simulink model "MdSWReqChk"  (R2024b)
settings: Solver=FixedStepDiscrete  StartTime=0.0  StopTime=10.0  FixedStep=0.01  RelTol=1e-3
undefined symbols (not defined in the file or in its folder): ChkBsyBitArray4s, ChkBsyBitArray6s7s, KeSMSAutoEZEFwdBkwdPosEna_Val, KeSMSuButtonLongPressedThrshldTm_Val, KeSMSuMdNum4s_Val, KeSMSuMdNum6s7s_Val, SetBsyBitArray4s, SetEnBitArray4s
libraries: simulink x16, RspLib x14
(part 3 of 3)

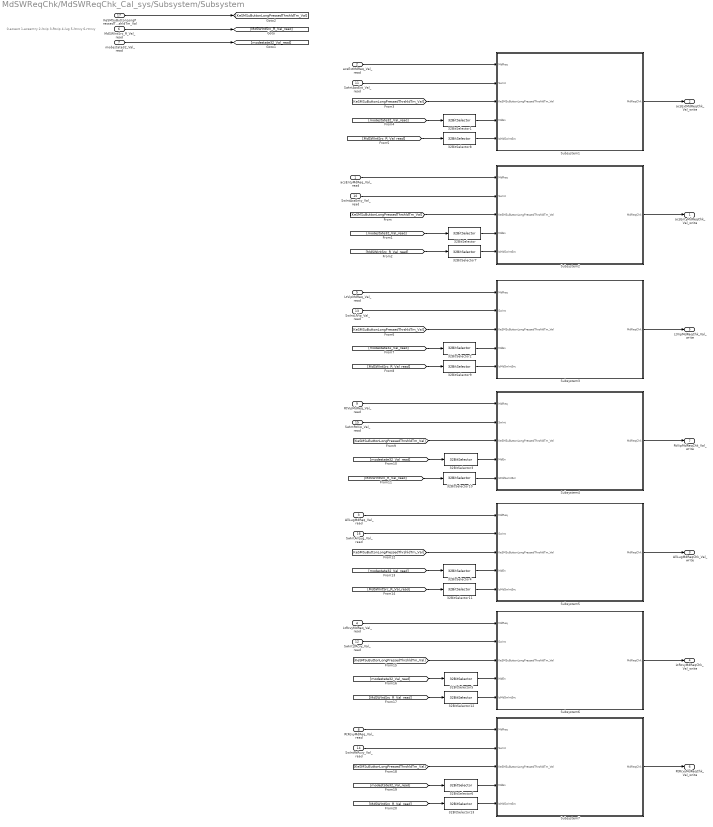
== system MdSWReqChk/MdSWReqChk_Cal_sys/Subsystem/Subsystem ==
  note: 0-acsext 1-acsentry 2-ltvip 3-Rtvip 4-lug 5-ltrcvy 6-rtrcvy
  acsEntyMdReq_Val_read : Inport
  acsExtMdReq_Val_read : Inport  Port=2
  AllLugMdReq_Val_read : Inport  Port=3
  LtRcvyMdReq_Val_read : Inport  Port=4
  LtVipMdReq_Val_read : Inport  Port=5
  MdSWIntSrc_R_Val_read : Inport  Port=6
  modestate32_Val_read : Inport  Port=7
  RtRcvyMdReq_Val_read : Inport  Port=8
  RtVipMdReq_Val_read : Inport  Port=9
  SwIntAcsEnty_Val_read : Inport  Port=10
  SwIntAcsExt_Val_read : Inport  Port=11
  SwIntLfRcvy_Val_read : Inport  Port=12
  SwIntLfVip_Val_read : Inport  Port=13
  SwIntRtRcvy_Val_read : Inport  Port=14
  SwIntRtVip_Val_read : Inport  Port=15
  SwIntAllLug_Val_read : Inport  Port=16
  KeSMSuButtonLongPressedThrshldTm_Val : Inport  Port=17
  32BitSelector : RspLib/32BitSelector  BitNum=0
  32BitSelector1 : RspLib/32BitSelector  BitNum=3
  32BitSelector10 : RspLib/32BitSelector  BitNum=3
  32BitSelector11 : RspLib/32BitSelector  BitNum=4
  32BitSelector12 : RspLib/32BitSelector  BitNum=5
  32BitSelector13 : RspLib/32BitSelector  BitNum=6
  32BitSelector2 : RspLib/32BitSelector  BitNum=9
  32BitSelector3 : RspLib/32BitSelector  BitNum=11
  32BitSelector4 : RspLib/32BitSelector  BitNum=2
  32BitSelector5 : RspLib/32BitSelector  BitNum=10
  32BitSelector6 : RspLib/32BitSelector  BitNum=12
  32BitSelector7 : RspLib/32BitSelector  BitNum=1
  32BitSelector8 : RspLib/32BitSelector  BitNum=0
  32BitSelector9 : RspLib/32BitSelector  BitNum=2
  Subsystem1 : Subsystem
  Subsystem2 : Subsystem
  Subsystem3 : Subsystem
  Subsystem4 : Subsystem
  Subsystem5 : Subsystem
  Subsystem6 : Subsystem
  Subsystem7 : Subsystem
  acsEntyMdReqChk_Val_write : Outport  VectorParamsAs1DForOutWhenUnconnected=off
      settings: EnsureOutportIsVirtual=on
  acsExtMdReqChk_Val_write : Outport  Port=2  VectorParamsAs1DForOutWhenUnconnected=off
      settings: EnsureOutportIsVirtual=on
  AllLugMdReqChk_Val_write : Outport  Port=3  VectorParamsAs1DForOutWhenUnconnected=off
      settings: EnsureOutportIsVirtual=on
  LtRcvyMdReqChk_Val_write : Outport  Port=4  VectorParamsAs1DForOutWhenUnconnected=off
      settings: EnsureOutportIsVirtual=on
  LtVipMdReqChk_Val_write : Outport  Port=5  VectorParamsAs1DForOutWhenUnconnected=off
      settings: EnsureOutportIsVirtual=on
  RtRcvyMdReqChk_Val_write : Outport  Port=6  VectorParamsAs1DForOutWhenUnconnected=off
      settings: EnsureOutportIsVirtual=on
  RtVipMdReqChk_Val_write : Outport  Port=7  VectorParamsAs1DForOutWhenUnconnected=off
      settings: EnsureOutportIsVirtual=on
  wires:
  modestate32_Val_read/1 -> [modestate32_Val_read]
  SwIntAcsExt_Val_read/1 -> Subsystem1/2(SwInt)
  MdSWIntSrc_R_Val_read/1 -> [MdSWIntSrc_R_Val_read]
  SwIntAcsEnty_Val_read/1 -> Subsystem2/2(SwInt)
  KeSMSuButtonLongPressedThrshldTm_Val/1 -> [KeSMSuButtonLongPressedThrshldTm_Val]
  [KeSMSuButtonLongPressedThrshldTm_Val] -> Subsystem2/3(KeSMSuButtonLongPressedThrshldTm_Val)
  [modestate32_Val_read] -> 32BitSelector/1
  32BitSelector/1 -> Subsystem2/4(MdEn)
  [MdSWIntSrc_R_Val_read] -> 32BitSelector7/1
  32BitSelector7/1 -> Subsystem2/5(IsMdSwIntSrc)
  Subsystem2/1(MdReqChk) -> acsEntyMdReqChk_Val_write/1
  [KeSMSuButtonLongPressedThrshldTm_Val] -> Subsystem1/3(KeSMSuButtonLongPressedThrshldTm_Val)
  32BitSelector1/1 -> Subsystem1/4(MdEn)
  [modestate32_Val_read] -> 32BitSelector1/1
  32BitSelector8/1 -> Subsystem1/5(IsMdSwIntSrc)
  [MdSWIntSrc_R_Val_read] -> 32BitSelector8/1
  Subsystem1/1(MdReqChk) -> acsExtMdReqChk_Val_write/1
  acsExtMdReq_Val_read/1 -> Subsystem1/1(MdReq)
  acsEntyMdReq_Val_read/1 -> Subsystem2/1(MdReq)
  32BitSelector2/1 -> Subsystem3/4(MdEn)
  32BitSelector9/1 -> Subsystem3/5(IsMdSwIntSrc)
  [KeSMSuButtonLongPressedThrshldTm_Val] -> Subsystem3/3(KeSMSuButtonLongPressedThrshldTm_Val)
  [modestate32_Val_read] -> 32BitSelector2/1
  32BitSelector3/1 -> Subsystem4/4(MdEn)
  32BitSelector10/1 -> Subsystem4/5(IsMdSwIntSrc)
  [KeSMSuButtonLongPressedThrshldTm_Val] -> Subsystem4/3(KeSMSuButtonLongPressedThrshldTm_Val)
  [modestate32_Val_read] -> 32BitSelector3/1
  32BitSelector4/1 -> Subsystem5/4(MdEn)
  32BitSelector11/1 -> Subsystem5/5(IsMdSwIntSrc)
  [KeSMSuButtonLongPressedThrshldTm_Val] -> Subsystem5/3(KeSMSuButtonLongPressedThrshldTm_Val)
  [modestate32_Val_read] -> 32BitSelector4/1
  32BitSelector5/1 -> Subsystem6/4(MdEn)
  32BitSelector12/1 -> Subsystem6/5(IsMdSwIntSrc)
  [KeSMSuButtonLongPressedThrshldTm_Val] -> Subsystem6/3(KeSMSuButtonLongPressedThrshldTm_Val)
  [modestate32_Val_read] -> 32BitSelector5/1
  32BitSelector6/1 -> Subsystem7/4(MdEn)
  32BitSelector13/1 -> Subsystem7/5(IsMdSwIntSrc)
  [KeSMSuButtonLongPressedThrshldTm_Val] -> Subsystem7/3(KeSMSuButtonLongPressedThrshldTm_Val)
  [modestate32_Val_read] -> 32BitSelector6/1
  LtVipMdReq_Val_read/1 -> Subsystem3/1(MdReq)
  SwIntLfVip_Val_read/1 -> Subsystem3/2(SwInt)
  SwIntRtVip_Val_read/1 -> Subsystem4/2(SwInt)
  RtVipMdReq_Val_read/1 -> Subsystem4/1(MdReq)
  AllLugMdReq_Val_read/1 -> Subsystem5/1(MdReq)
  SwIntLfRcvy_Val_read/1 -> Subsystem6/2(SwInt)
  SwIntRtRcvy_Val_read/1 -> Subsystem7/2(SwInt)
  LtRcvyMdReq_Val_read/1 -> Subsystem6/1(MdReq)
  RtRcvyMdReq_Val_read/1 -> Subsystem7/1(MdReq)
  Subsystem3/1(MdReqChk) -> LtVipMdReqChk_Val_write/1
  Subsystem4/1(MdReqChk) -> RtVipMdReqChk_Val_write/1
  Subsystem5/1(MdReqChk) -> AllLugMdReqChk_Val_write/1
  Subsystem6/1(MdReqChk) -> LtRcvyMdReqChk_Val_write/1
  Subsystem7/1(MdReqChk) -> RtRcvyMdReqChk_Val_write/1
  SwIntAllLug_Val_read/1 -> Subsystem5/2(SwInt)
  [MdSWIntSrc_R_Val_read] -> 32BitSelector9/1
  [MdSWIntSrc_R_Val_read] -> 32BitSelector10/1
  [MdSWIntSrc_R_Val_read] -> 32BitSelector11/1
  [MdSWIntSrc_R_Val_read] -> 32BitSelector12/1
  [MdSWIntSrc_R_Val_read] -> 32BitSelector13/1

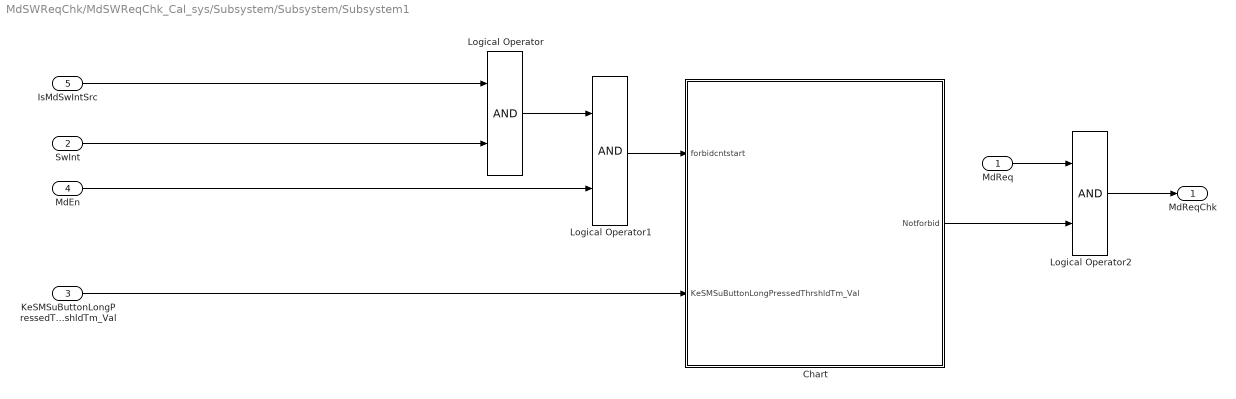
== system MdSWReqChk/MdSWReqChk_Cal_sys/Subsystem/Subsystem/Subsystem1 ==
  MdReq : Inport
  SwInt : Inport  Port=2
  KeSMSuButtonLongPressedThrshldTm_Val : Inport  Port=3
  MdEn : Inport  Port=4
  IsMdSwIntSrc : Inport  Port=5
  Chart : Stateflow chart  TreatAsAtomicUnit=on
  Logical Operator : Logic  AllPortsSameDT=off  OutDataTypeStr=boolean
  Logical Operator1 : Logic  AllPortsSameDT=off  OutDataTypeStr=boolean
  Logical Operator2 : Logic  AllPortsSameDT=off  OutDataTypeStr=boolean
  MdReqChk : Outport  VectorParamsAs1DForOutWhenUnconnected=off
  wires:
  KeSMSuButtonLongPressedThrshldTm_Val/1 -> Chart/2(KeSMSuButtonLongPressedThrshldTm_Val)
  Logical Operator1/1 -> Chart/1(forbidcntstart)
  MdEn/1 -> Logical Operator1/2
  Logical Operator/1 -> Logical Operator1/1
  SwInt/1 -> Logical Operator/2
  IsMdSwIntSrc/1 -> Logical Operator/1
  Chart/1(Notforbid) -> Logical Operator2/2
  MdReq/1 -> Logical Operator2/1
  Logical Operator2/1 -> MdReqChk/1

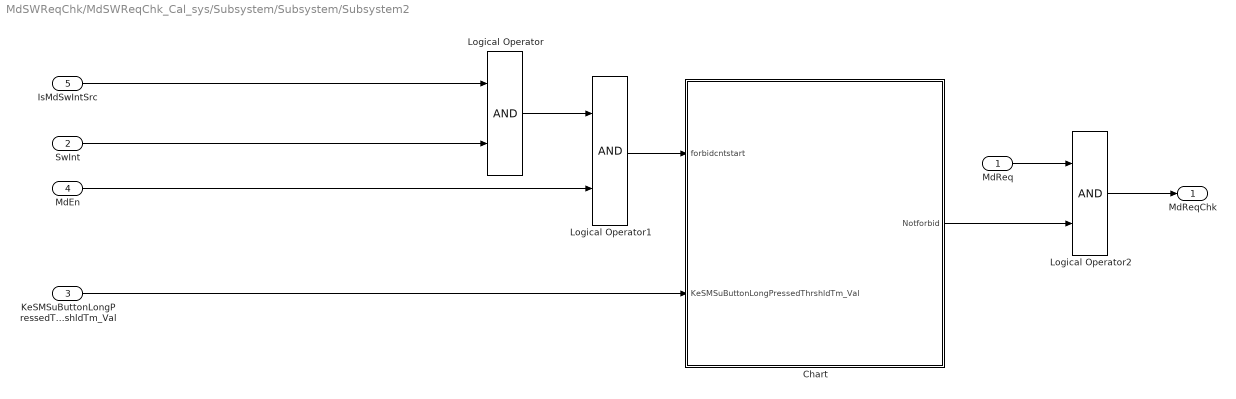
== system MdSWReqChk/MdSWReqChk_Cal_sys/Subsystem/Subsystem/Subsystem2 ==
  MdReq : Inport
  SwInt : Inport  Port=2
  KeSMSuButtonLongPressedThrshldTm_Val : Inport  Port=3
  MdEn : Inport  Port=4
  IsMdSwIntSrc : Inport  Port=5
  Chart : Stateflow chart  TreatAsAtomicUnit=on
  Logical Operator : Logic  AllPortsSameDT=off  OutDataTypeStr=boolean
  Logical Operator1 : Logic  AllPortsSameDT=off  OutDataTypeStr=boolean
  Logical Operator2 : Logic  AllPortsSameDT=off  OutDataTypeStr=boolean
  MdReqChk : Outport  VectorParamsAs1DForOutWhenUnconnected=off
  wires:
  Logical Operator2/1 -> MdReqChk/1
  MdReq/1 -> Logical Operator2/1
  Chart/1(Notforbid) -> Logical Operator2/2
  IsMdSwIntSrc/1 -> Logical Operator/1
  SwInt/1 -> Logical Operator/2
  Logical Operator/1 -> Logical Operator1/1
  MdEn/1 -> Logical Operator1/2
  Logical Operator1/1 -> Chart/1(forbidcntstart)
  KeSMSuButtonLongPressedThrshldTm_Val/1 -> Chart/2(KeSMSuButtonLongPressedThrshldTm_Val)

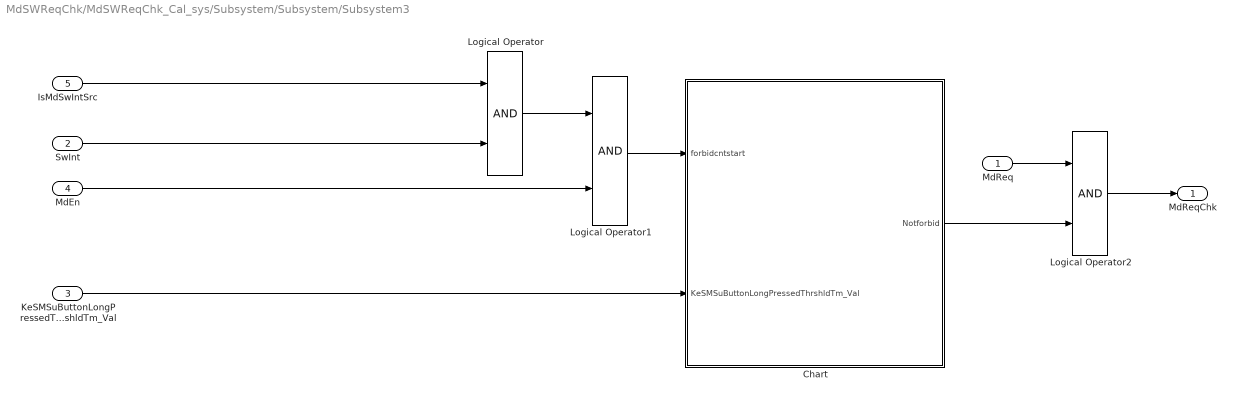
== system MdSWReqChk/MdSWReqChk_Cal_sys/Subsystem/Subsystem/Subsystem3 ==
  MdReq : Inport
  SwInt : Inport  Port=2
  KeSMSuButtonLongPressedThrshldTm_Val : Inport  Port=3
  MdEn : Inport  Port=4
  IsMdSwIntSrc : Inport  Port=5
  Chart : Stateflow chart  TreatAsAtomicUnit=on
  Logical Operator : Logic  AllPortsSameDT=off  OutDataTypeStr=boolean
  Logical Operator1 : Logic  AllPortsSameDT=off  OutDataTypeStr=boolean
  Logical Operator2 : Logic  AllPortsSameDT=off  OutDataTypeStr=boolean
  MdReqChk : Outport  VectorParamsAs1DForOutWhenUnconnected=off
  wires:
  Logical Operator2/1 -> MdReqChk/1
  MdReq/1 -> Logical Operator2/1
  Chart/1(Notforbid) -> Logical Operator2/2
  IsMdSwIntSrc/1 -> Logical Operator/1
  SwInt/1 -> Logical Operator/2
  Logical Operator/1 -> Logical Operator1/1
  MdEn/1 -> Logical Operator1/2
  Logical Operator1/1 -> Chart/1(forbidcntstart)
  KeSMSuButtonLongPressedThrshldTm_Val/1 -> Chart/2(KeSMSuButtonLongPressedThrshldTm_Val)

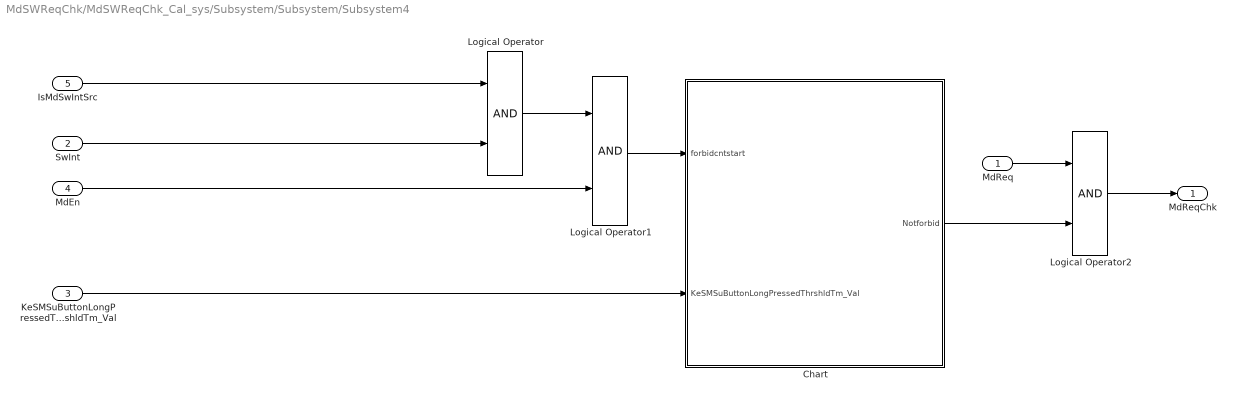
== system MdSWReqChk/MdSWReqChk_Cal_sys/Subsystem/Subsystem/Subsystem4 ==
  MdReq : Inport
  SwInt : Inport  Port=2
  KeSMSuButtonLongPressedThrshldTm_Val : Inport  Port=3
  MdEn : Inport  Port=4
  IsMdSwIntSrc : Inport  Port=5
  Chart : Stateflow chart  TreatAsAtomicUnit=on
  Logical Operator : Logic  AllPortsSameDT=off  OutDataTypeStr=boolean
  Logical Operator1 : Logic  AllPortsSameDT=off  OutDataTypeStr=boolean
  Logical Operator2 : Logic  AllPortsSameDT=off  OutDataTypeStr=boolean
  MdReqChk : Outport  VectorParamsAs1DForOutWhenUnconnected=off
  wires:
  KeSMSuButtonLongPressedThrshldTm_Val/1 -> Chart/2(KeSMSuButtonLongPressedThrshldTm_Val)
  Logical Operator1/1 -> Chart/1(forbidcntstart)
  MdEn/1 -> Logical Operator1/2
  Logical Operator/1 -> Logical Operator1/1
  SwInt/1 -> Logical Operator/2
  IsMdSwIntSrc/1 -> Logical Operator/1
  Chart/1(Notforbid) -> Logical Operator2/2
  MdReq/1 -> Logical Operator2/1
  Logical Operator2/1 -> MdReqChk/1

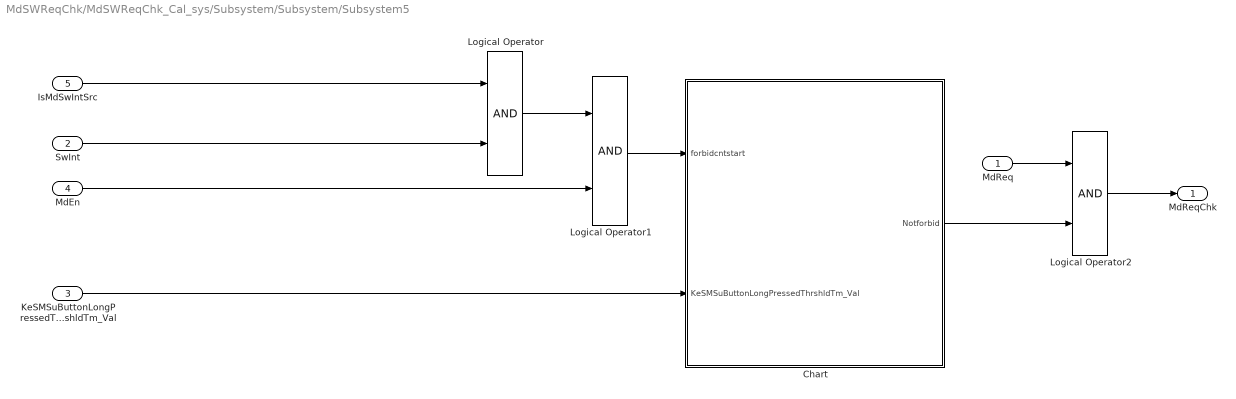
== system MdSWReqChk/MdSWReqChk_Cal_sys/Subsystem/Subsystem/Subsystem5 ==
  MdReq : Inport
  SwInt : Inport  Port=2
  KeSMSuButtonLongPressedThrshldTm_Val : Inport  Port=3
  MdEn : Inport  Port=4
  IsMdSwIntSrc : Inport  Port=5
  Chart : Stateflow chart  TreatAsAtomicUnit=on
  Logical Operator : Logic  AllPortsSameDT=off  OutDataTypeStr=boolean
  Logical Operator1 : Logic  AllPortsSameDT=off  OutDataTypeStr=boolean
  Logical Operator2 : Logic  AllPortsSameDT=off  OutDataTypeStr=boolean
  MdReqChk : Outport  VectorParamsAs1DForOutWhenUnconnected=off
  wires:
  Logical Operator2/1 -> MdReqChk/1
  MdReq/1 -> Logical Operator2/1
  Chart/1(Notforbid) -> Logical Operator2/2
  IsMdSwIntSrc/1 -> Logical Operator/1
  SwInt/1 -> Logical Operator/2
  Logical Operator/1 -> Logical Operator1/1
  MdEn/1 -> Logical Operator1/2
  Logical Operator1/1 -> Chart/1(forbidcntstart)
  KeSMSuButtonLongPressedThrshldTm_Val/1 -> Chart/2(KeSMSuButtonLongPressedThrshldTm_Val)

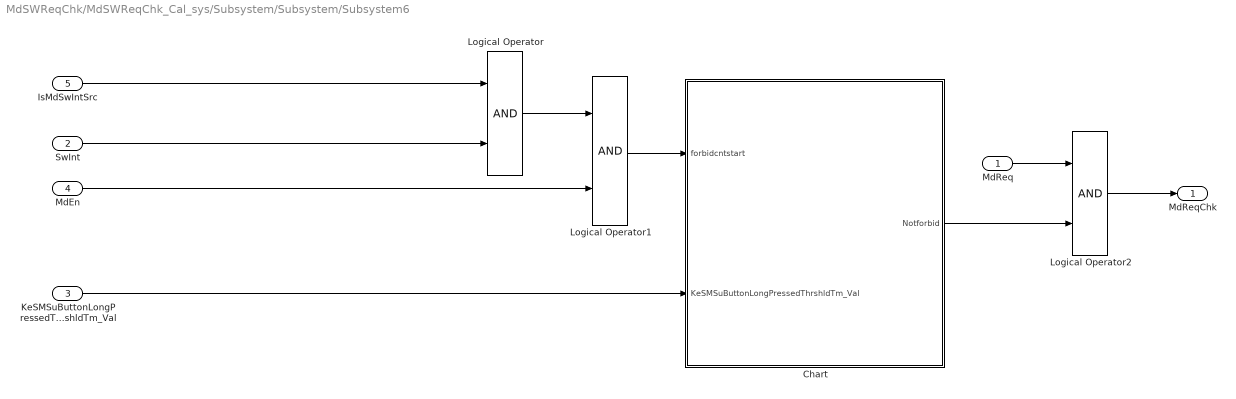
== system MdSWReqChk/MdSWReqChk_Cal_sys/Subsystem/Subsystem/Subsystem6 ==
  MdReq : Inport
  SwInt : Inport  Port=2
  KeSMSuButtonLongPressedThrshldTm_Val : Inport  Port=3
  MdEn : Inport  Port=4
  IsMdSwIntSrc : Inport  Port=5
  Chart : Stateflow chart  TreatAsAtomicUnit=on
  Logical Operator : Logic  AllPortsSameDT=off  OutDataTypeStr=boolean
  Logical Operator1 : Logic  AllPortsSameDT=off  OutDataTypeStr=boolean
  Logical Operator2 : Logic  AllPortsSameDT=off  OutDataTypeStr=boolean
  MdReqChk : Outport  VectorParamsAs1DForOutWhenUnconnected=off
  wires:
  KeSMSuButtonLongPressedThrshldTm_Val/1 -> Chart/2(KeSMSuButtonLongPressedThrshldTm_Val)
  Logical Operator1/1 -> Chart/1(forbidcntstart)
  MdEn/1 -> Logical Operator1/2
  Logical Operator/1 -> Logical Operator1/1
  SwInt/1 -> Logical Operator/2
  IsMdSwIntSrc/1 -> Logical Operator/1
  Chart/1(Notforbid) -> Logical Operator2/2
  MdReq/1 -> Logical Operator2/1
  Logical Operator2/1 -> MdReqChk/1

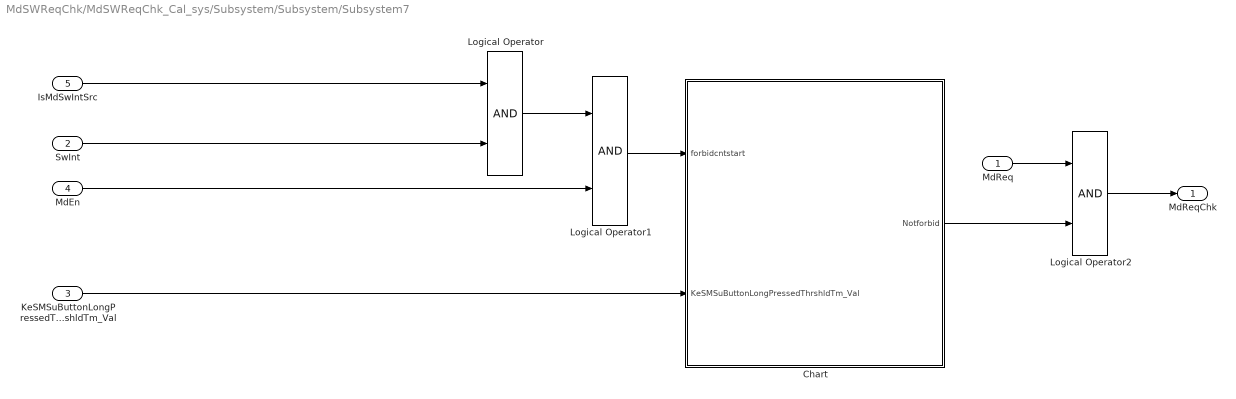
== system MdSWReqChk/MdSWReqChk_Cal_sys/Subsystem/Subsystem/Subsystem7 ==
  MdReq : Inport
  SwInt : Inport  Port=2
  KeSMSuButtonLongPressedThrshldTm_Val : Inport  Port=3
  MdEn : Inport  Port=4
  IsMdSwIntSrc : Inport  Port=5
  Chart : Stateflow chart  TreatAsAtomicUnit=on
  Logical Operator : Logic  AllPortsSameDT=off  OutDataTypeStr=boolean
  Logical Operator1 : Logic  AllPortsSameDT=off  OutDataTypeStr=boolean
  Logical Operator2 : Logic  AllPortsSameDT=off  OutDataTypeStr=boolean
  MdReqChk : Outport  VectorParamsAs1DForOutWhenUnconnected=off
  wires:
  Logical Operator2/1 -> MdReqChk/1
  MdReq/1 -> Logical Operator2/1
  Chart/1(Notforbid) -> Logical Operator2/2
  IsMdSwIntSrc/1 -> Logical Operator/1
  SwInt/1 -> Logical Operator/2
  Logical Operator/1 -> Logical Operator1/1
  MdEn/1 -> Logical Operator1/2
  Logical Operator1/1 -> Chart/1(forbidcntstart)
  KeSMSuButtonLongPressedThrshldTm_Val/1 -> Chart/2(KeSMSuButtonLongPressedThrshldTm_Val)

== stateflow chart MdSWReqChk/MdSWReqChk_Cal_sys/Subsystem/Subsystem/Subsystem1/Chart ==
  state fobidStop
    en:Notforbid = true;
  state fobidCntStart
    en:forbidcnt=1;
    du:forbidcnt=forbidcnt+1;
  state fobid
    en:Notforbid=false;
    en:forbidcnt=1;
    du:forbidcnt=forbidcnt+1;
  (default) -> fobidStop
  fobidStop -> fobidCntStart : [forbidcntstart]
  fobidCntStart -> fobid : [forbidcnt>=(KeSMSuButtonLongPressedThrshldTm_Val-5)]
  fobid -> fobidStop : [forbidcnt >10]
  data: forbidcntstart input boolean; forbidcnt local uint8; KeSMSuButtonLongPressedThrshldTm_Val input; Notforbid output boolean

== stateflow chart MdSWReqChk/MdSWReqChk_Cal_sys/Subsystem/Subsystem/Subsystem2/Chart ==
  state fobidStop
    en:Notforbid = true;
  state fobidCntStart
    en:forbidcnt=1;
    du:forbidcnt=forbidcnt+1;
  state fobid
    en:Notforbid=false;
    en:forbidcnt=1;
    du:forbidcnt=forbidcnt+1;
  (default) -> fobidStop
  fobidStop -> fobidCntStart : [forbidcntstart]
  fobidCntStart -> fobid : [forbidcnt>=(KeSMSuButtonLongPressedThrshldTm_Val-5)]
  fobid -> fobidStop : [forbidcnt >10]
  data: forbidcntstart input boolean; forbidcnt local uint8; KeSMSuButtonLongPressedThrshldTm_Val input; Notforbid output boolean

== stateflow chart MdSWReqChk/MdSWReqChk_Cal_sys/Subsystem/Subsystem/Subsystem3/Chart ==
  state fobidStop
    en:Notforbid = true;
  state fobidCntStart
    en:forbidcnt=1;
    du:forbidcnt=forbidcnt+1;
  state fobid
    en:Notforbid=false;
    en:forbidcnt=1;
    du:forbidcnt=forbidcnt+1;
  (default) -> fobidStop
  fobidStop -> fobidCntStart : [forbidcntstart]
  fobidCntStart -> fobid : [forbidcnt>=(KeSMSuButtonLongPressedThrshldTm_Val-5)]
  fobid -> fobidStop : [forbidcnt >10]
  data: forbidcntstart input boolean; forbidcnt local uint8; KeSMSuButtonLongPressedThrshldTm_Val input; Notforbid output boolean

== stateflow chart MdSWReqChk/MdSWReqChk_Cal_sys/Subsystem/Subsystem/Subsystem4/Chart ==
  state fobidStop
    en:Notforbid = true;
  state fobidCntStart
    en:forbidcnt=1;
    du:forbidcnt=forbidcnt+1;
  state fobid
    en:Notforbid=false;
    en:forbidcnt=1;
    du:forbidcnt=forbidcnt+1;
  (default) -> fobidStop
  fobidStop -> fobidCntStart : [forbidcntstart]
  fobidCntStart -> fobid : [forbidcnt>=(KeSMSuButtonLongPressedThrshldTm_Val-5)]
  fobid -> fobidStop : [forbidcnt >10]
  data: forbidcntstart input boolean; forbidcnt local uint8; KeSMSuButtonLongPressedThrshldTm_Val input; Notforbid output boolean

== stateflow chart MdSWReqChk/MdSWReqChk_Cal_sys/Subsystem/Subsystem/Subsystem5/Chart ==
  state fobidStop
    en:Notforbid = true;
  state fobidCntStart
    en:forbidcnt=1;
    du:forbidcnt=forbidcnt+1;
  state fobid
    en:Notforbid=false;
    en:forbidcnt=1;
    du:forbidcnt=forbidcnt+1;
  (default) -> fobidStop
  fobidStop -> fobidCntStart : [forbidcntstart]
  fobidCntStart -> fobid : [forbidcnt>=(KeSMSuButtonLongPressedThrshldTm_Val-5)]
  fobid -> fobidStop : [forbidcnt >10]
  data: forbidcntstart input boolean; forbidcnt local uint8; KeSMSuButtonLongPressedThrshldTm_Val input; Notforbid output boolean

== stateflow chart MdSWReqChk/MdSWReqChk_Cal_sys/Subsystem/Subsystem/Subsystem6/Chart ==
  state fobidStop
    en:Notforbid = true;
  state fobidCntStart
    en:forbidcnt=1;
    du:forbidcnt=forbidcnt+1;
  state fobid
    en:Notforbid=false;
    en:forbidcnt=1;
    du:forbidcnt=forbidcnt+1;
  (default) -> fobidStop
  fobidStop -> fobidCntStart : [forbidcntstart]
  fobidCntStart -> fobid : [forbidcnt>=(KeSMSuButtonLongPressedThrshldTm_Val-5)]
  fobid -> fobidStop : [forbidcnt >10]
  data: forbidcntstart input boolean; forbidcnt local uint8; KeSMSuButtonLongPressedThrshldTm_Val input; Notforbid output boolean

== stateflow chart MdSWReqChk/MdSWReqChk_Cal_sys/Subsystem/Subsystem/Subsystem7/Chart ==
  state fobidStop
    en:Notforbid = true;
  state fobidCntStart
    en:forbidcnt=1;
    du:forbidcnt=forbidcnt+1;
  state fobid
    en:Notforbid=false;
    en:forbidcnt=1;
    du:forbidcnt=forbidcnt+1;
  (default) -> fobidStop
  fobidStop -> fobidCntStart : [forbidcntstart]
  fobidCntStart -> fobid : [forbidcnt>=(KeSMSuButtonLongPressedThrshldTm_Val-5)]
  fobid -> fobidStop : [forbidcnt >10]
  data: forbidcntstart input boolean; forbidcnt local uint8; KeSMSuButtonLongPressedThrshldTm_Val input; Notforbid output boolean
